simulink model "Mruti_Dz_Mathematical_modeling"  (R2023b)
settings: Solver=VariableStepAuto  StartTime=0.0  StopTime=10.0  RelTol=1e-3
undefined symbols (not defined in the file): magnitude
libraries: simulink x1
settings Model: Creator=HP5CD  LastModifiedBy=HP5CD

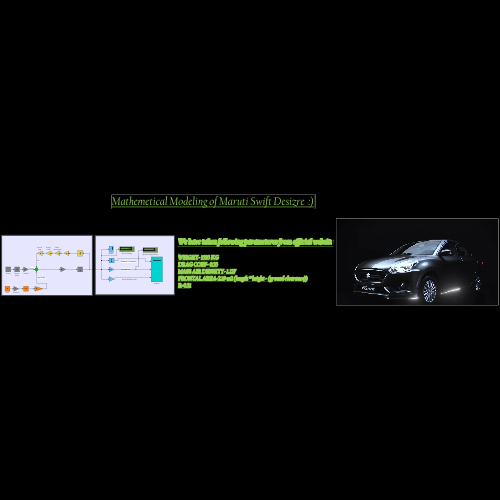
[thumbnail: Simulink's stored preview of the top-level diagram]
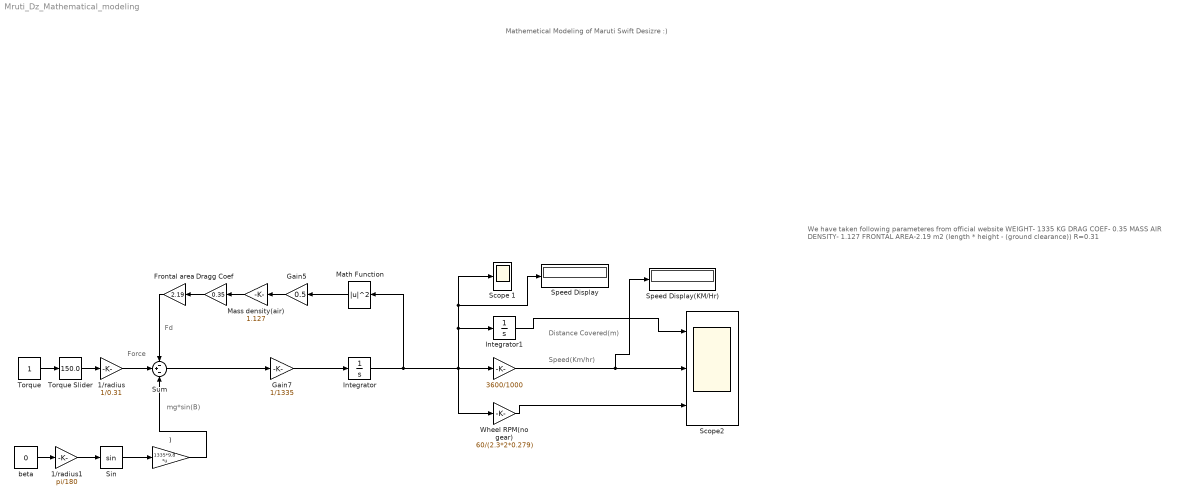
== system Mruti_Dz_Mathematical_modeling ==
  note: We have taken following parameteres from official website
      |
      | WEIGHT- 1335 KG
      | DRAG COEF- 0.35
      | MASS AIR DENSITY- 1.127
      | FRONTAL AREA-2.19 m2 (length * height - (ground clearance))
      | R=0.31
  note: Mathemetical Modeling of Maruti Swift Desizre :)
  note: mg*sin(B)
  note: Fd
  note: Distance Covered(m)
  note: Force
  note: Speed(Km/hr)
  "                " : Gain  Gain=3600/1000
  "                Wheel RPM(no gear)" : Gain  Gain=60/(2.3*2*0.279)
  ) : Gain  Gain=1335*9.8  Multiplication=Matrix(K*u)
  1/radius : Gain  Gain=1/0.31
  1/radius1 : Gain  Gain=pi/180
  Dragg Coef : Gain  Gain=0.35
  Frontal area : Gain  Gain=2.19
  Gain5 : Gain  Gain=0.5
  Gain7 : Gain  Gain=1/1335
  Integrator : Integrator
  Integrator1 : Integrator
  Mass density(air) : Gain  Gain=1.127
  Math Function : Math  Operator=magnitude^2
  Scope 1 : Scope
  Scope2 : Scope  NumInputPorts=3
  Sin : Trigonometry
  Speed Display : Display
  Speed Display(KM/Hr) : Display
  Sum : Sum  Inputs=-+-
  Torque : Constant
  Torque Slider : simulink/Math Operations/Slider Gain  gain=150.0  low=100  high=150
  beta : Constant  Value=0
  wires:
  1/radius1/1 -> Sin/1
  "                "/1 -> Speed Display(KM/Hr)/1, Scope2/2
  "                Wheel RPM(no gear)"/1 -> Scope2/3
  Torque Slider/1 -> 1/radius/1
  Frontal area/1 -> Sum/1
  Mass density(air)/1 -> Dragg Coef/1
  Sin/1 -> )/1
  Torque/1 -> Torque Slider/1
  Integrator1/1 -> Scope2/1
  Integrator/1 -> Integrator1/1, Speed Display/1, Scope 1/1, "                "/1, "                Wheel RPM(no gear)"/1, Math Function/1
  )/1 -> Sum/3
  Sum/1 -> Gain7/1
  beta/1 -> 1/radius1/1
  1/radius/1 -> Sum/2
  Gain5/1 -> Mass density(air)/1
  Math Function/1 -> Gain5/1
  Dragg Coef/1 -> Frontal area/1
  Gain7/1 -> Integrator/1
